simulink model "Trajectory_generation"  (R2020b)
settings: Solver=VariableStepAuto  StartTime=0.0  StopTime=16  RelTol=1e-3
values from neighbouring files (symbols this model uses):
  deltaS = deltaS_values(index)    [trajectory_generation.m]
  Vx_final = 40    [trajectory_generation.m]
  Vy_final = 0    [trajectory_generation.m]
  Vz_final = 0    [trajectory_generation.m]
  x_final = 500    [trajectory_generation.m]
  y_final = 0    [trajectory_generation.m]
  z_final = 1300    [trajectory_generation.m]
settings Model: Creator=adm-w10  LastModifiedBy=aless
settings SFSimCC: CustomCodeUndefinedFunction=UseInterfaceOnly

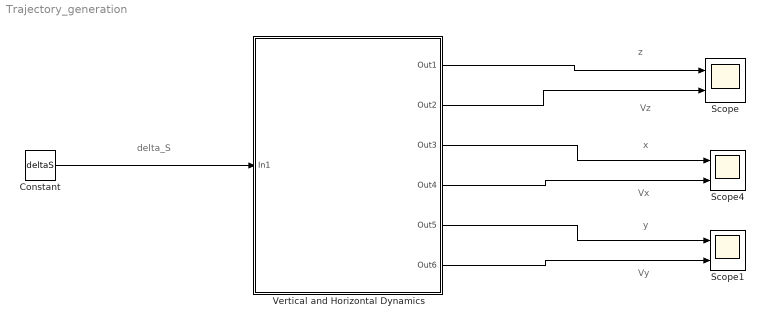
== system Trajectory_generation ==
  note: delta_S
  note: Vz
  note: z
  note: Vx
  note: x
  note: Vy
  note: y
  Constant : Constant  Value=deltaS
  Scope : Scope  NumInputPorts=2
  Scope1 : Scope  NumInputPorts=2
  Scope4 : Scope  NumInputPorts=2
  Vertical and Horizontal Dynamics : Subsystem
  wires:
  Constant/1 -> Vertical and Horizontal Dynamics/1(In1)
  Vertical and Horizontal Dynamics/3(Out3) -> Scope4/1
  Vertical and Horizontal Dynamics/4(Out4) -> Scope4/2
  Vertical and Horizontal Dynamics/1(Out1) -> Scope/1
  Vertical and Horizontal Dynamics/2(Out2) -> Scope/2
  Vertical and Horizontal Dynamics/5(Out5) -> Scope1/1
  Vertical and Horizontal Dynamics/6(Out6) -> Scope1/2

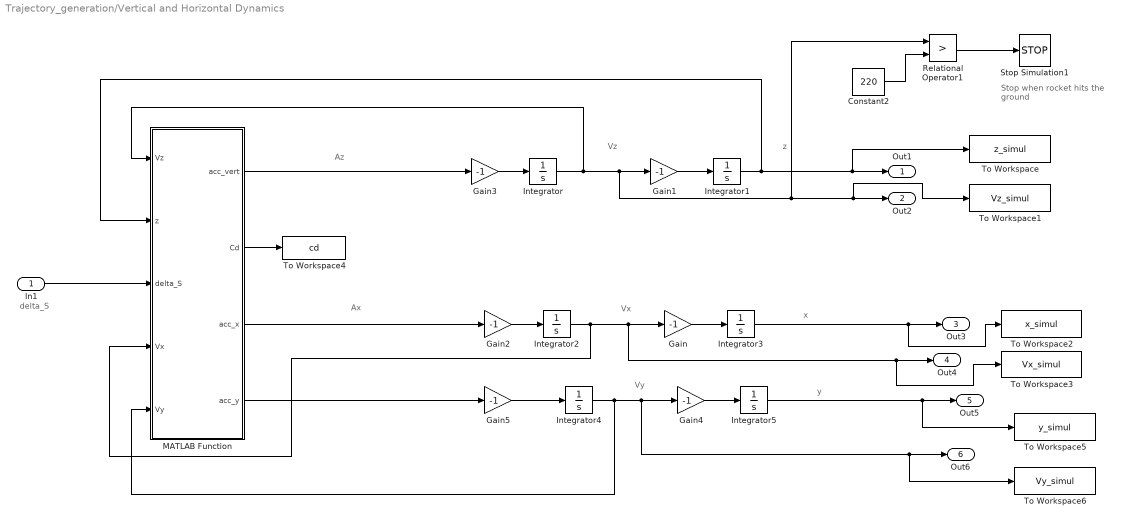
== system Trajectory_generation/Vertical and Horizontal Dynamics ==
  note: x
  note: delta_S
  note: Az
  note: Vz
  note: z
  note: Ax
  note: Vx
  note: Stop when rocket
      |  hits the ground
  note: y
  note: Vy
  In1 : Inport
  Constant2 : Constant  Value=220
  Gain{,1..5} (6 alike) : Gain  Gain=-1
  Integrator : Integrator  InitialCondition=Vz_final
  Integrator1 : Integrator  InitialCondition=z_final
  Integrator2 : Integrator  InitialCondition=Vx_final
  Integrator3 : Integrator  InitialCondition=x_final
  Integrator4 : Integrator  InitialCondition=Vy_final
  Integrator5 : Integrator  InitialCondition=y_final
  MATLAB Function : MATLAB Function  TreatAsAtomicUnit=on  SystemSampleTime=0.05
  Relational Operator1 : RelationalOperator  Operator=>  OutDataTypeStr=boolean  RndMeth=Simplest
  Stop Simulation1 : Stop
  To Workspace : ToWorkspace  VariableName=z_simul  SampleTime=-1
  To Workspace1 : ToWorkspace  VariableName=Vz_simul  SampleTime=-1
  To Workspace2 : ToWorkspace  VariableName=x_simul  SampleTime=-1
  To Workspace3 : ToWorkspace  VariableName=Vx_simul  SampleTime=-1
  To Workspace4 : ToWorkspace  VariableName=cd  SampleTime=-1
  To Workspace5 : ToWorkspace  VariableName=y_simul  SampleTime=-1
  To Workspace6 : ToWorkspace  VariableName=Vy_simul  SampleTime=-1
  Out1 : Outport  VectorParamsAs1DForOutWhenUnconnected=off
  Out2 : Outport  Port=2  VectorParamsAs1DForOutWhenUnconnected=off
  Out3 : Outport  Port=3  VectorParamsAs1DForOutWhenUnconnected=off
  Out4 : Outport  Port=4  VectorParamsAs1DForOutWhenUnconnected=off
  Out5 : Outport  Port=5  VectorParamsAs1DForOutWhenUnconnected=off
  Out6 : Outport  Port=6  VectorParamsAs1DForOutWhenUnconnected=off
  wires:
  In1/1 -> MATLAB Function/3(delta_S)
  MATLAB Function/1(acc_vert) -> Gain3/1
  Integrator/1 -> MATLAB Function/1(Vz), Gain1/1, Relational Operator1/1, To Workspace1/1, Out2/1
  MATLAB Function/3(acc_x) -> Gain2/1
  Integrator2/1 -> To Workspace3/1, Out4/1, Gain/1, MATLAB Function/4(Vx)
  Integrator3/1 -> To Workspace2/1, Out3/1
  Gain1/1 -> Integrator1/1
  Gain/1 -> Integrator3/1
  Gain2/1 -> Integrator2/1
  Gain3/1 -> Integrator/1
  Integrator1/1 -> MATLAB Function/2(z), To Workspace/1, Out1/1
  MATLAB Function/2(Cd) -> To Workspace4/1
  Relational Operator1/1 -> Stop Simulation1/1
  Constant2/1 -> Relational Operator1/2
  Gain4/1 -> Integrator5/1
  MATLAB Function/4(acc_y) -> Gain5/1
  Integrator4/1 -> MATLAB Function/5(Vy), To Workspace6/1, Out6/1, Gain4/1
  Gain5/1 -> Integrator4/1
  Integrator5/1 -> To Workspace5/1, Out5/1

== matlab function Trajectory_generation/Vertical and Horizontal Dynamics/MATLAB Function ==
  data: Vz input; z input; delta_S input; acc_vert output; Cd output; acc_x output; Vx input; Vy input; acc_y output
function [acc_vert, Cd, acc_x, acc_y] = model( Vz, z, delta_S, Vx, Vy )  

% Necessary to compute Cd
data=load('coeffs.mat');

% Parameters
ro = getRho(z);
m = 19.20;  
g = 9.81;
diameter = 0.15; 
S0 = (pi*diameter^2)/4; 

% Compute the modulus of velocity
V_mod = sqrt(Vx^2+Vz^2+Vy^2);

% Obtain the Cd value ( It includes also the airbrake surface )
Cd = getDrag(V_mod,z,delta_S, data.coeffs);

% Compute the vertical and horizontal accelerations using the dynamic equations
acc_vert  = (-0.5*ro*S0*Cd*Vz*V_mod - m*g)/m;
acc_x = (-0.5*ro*S0*Cd*Vx*V_mod)/m;
acc_y = (-0.5*ro*S0*Cd*Vy*V_mod)/m;

end
